simulink model "HANcoder_E407_TTA_Controller_v4_6"  (R2018b)
settings: Solver=FixedStepDiscrete  StartTime=0.0  StopTime=1  FixedStep=0.01  RelTol=1e-3
PreLoadFcn:
  | librarySetup
  | eval([bdroot,'_startup']) %Calling [modelName]_startup.m
values from neighbouring files (symbols this model uses):
  Backup_Board = 0    [HANcoder_E407_TTA_Controller_v3_5_startup.m]    (also in HANcoder_E407_TTA_Controller_v4_6_startup.m; HANcoder_E407_TTA_Controller_v4_7_startup.m; HANcoder_E407_TTA_Controller_v4_startup.m)
  basic_cycle_duration_bc0 = TM_Reset_Board   + COMP_duration    (= 212)    [HANcoder_E407_TTA_Controller_v3_5_startup.m]    (also in HANcoder_E407_TTA_Controller_v4_6_startup.m; HANcoder_E407_TTA_Controller_v4_7_startup.m; HANcoder_E407_TTA_Controller_v4_startup.m)
  basic_cycle_duration_bc1 = TM_Reset_Var_bc1 + COMP_duration    (= 288)    [HANcoder_E407_TTA_Controller_v3_5_startup.m]    (also in HANcoder_E407_TTA_Controller_v4_6_startup.m = 332; HANcoder_E407_TTA_Controller_v4_7_startup.m = 372; HANcoder_E407_TTA_Controller_v4_startup.m = 332)
  comm_delay_estimation1 = round(comm_delay_measured1*hardware_granularity/frequency_IRQ)    [HANcoder_E407_TTA_Controller_v3_5_startup.m]    (also in HANcoder_E407_TTA_Controller_v4_6_startup.m; HANcoder_E407_TTA_Controller_v4_7_startup.m; HANcoder_E407_TTA_Controller_v4_startup.m)
  comm_delay_estimation2 = round(comm_delay_measured2*hardware_granularity/frequency_IRQ)    [HANcoder_E407_TTA_Controller_v3_5_startup.m]    (also in HANcoder_E407_TTA_Controller_v4_6_startup.m; HANcoder_E407_TTA_Controller_v4_7_startup.m; HANcoder_E407_TTA_Controller_v4_startup.m)
  COMM_Period = 40    [HANcoder_E407_TTA_Controller_v3_5_startup.m]    (also in HANcoder_E407_TTA_Controller_v4_6_startup.m; HANcoder_E407_TTA_Controller_v4_7_startup.m; HANcoder_E407_TTA_Controller_v4_startup.m)
  COMM_Phase1 = Simulink.Parameter    [HANcoder_E407_TTA_Controller_v3_5_startup.m]    (also in HANcoder_E407_TTA_Controller_v4_6_startup.m; HANcoder_E407_TTA_Controller_v4_7_startup.m; HANcoder_E407_TTA_Controller_v4_startup.m)
  COMM_Phase2 = Simulink.Parameter    [HANcoder_E407_TTA_Controller_v3_5_startup.m]    (also in HANcoder_E407_TTA_Controller_v4_6_startup.m; HANcoder_E407_TTA_Controller_v4_7_startup.m; HANcoder_E407_TTA_Controller_v4_startup.m)
  COMM_Phase_init1 = Simulink.Parameter    [HANcoder_E407_TTA_Controller_v3_5_startup.m]    (also in HANcoder_E407_TTA_Controller_v4_6_startup.m; HANcoder_E407_TTA_Controller_v4_7_startup.m; HANcoder_E407_TTA_Controller_v4_startup.m)
  COMM_Phase_init2 = Simulink.Parameter    [HANcoder_E407_TTA_Controller_v3_5_startup.m]    (also in HANcoder_E407_TTA_Controller_v4_6_startup.m; HANcoder_E407_TTA_Controller_v4_7_startup.m; HANcoder_E407_TTA_Controller_v4_startup.m)
  COMP_duration = 4    [HANcoder_E407_TTA_Controller_v3_5_startup.m]    (also in HANcoder_E407_TTA_Controller_v4_6_startup.m; HANcoder_E407_TTA_Controller_v4_7_startup.m; HANcoder_E407_TTA_Controller_v4_startup.m)
  Controller1_Board = 1    [HANcoder_E407_TTA_Controller_v3_5_startup.m]    (also in HANcoder_E407_TTA_Controller_v4_6_startup.m; HANcoder_E407_TTA_Controller_v4_7_startup.m; HANcoder_E407_TTA_Controller_v4_startup.m)
  Controller2_Board = 2    [HANcoder_E407_TTA_Controller_v3_5_startup.m]    (also in HANcoder_E407_TTA_Controller_v4_6_startup.m; HANcoder_E407_TTA_Controller_v4_7_startup.m; HANcoder_E407_TTA_Controller_v4_startup.m)
  Controller3_Board = 3    [HANcoder_E407_TTA_Controller_v3_5_startup.m]    (also in HANcoder_E407_TTA_Controller_v4_6_startup.m; HANcoder_E407_TTA_Controller_v4_7_startup.m; HANcoder_E407_TTA_Controller_v4_startup.m)
  delta_a_set = Simulink.Parameter    [HANcoder_E407_TTA_Controller_v3_5_startup.m]    (also in HANcoder_E407_TTA_Controller_v4_6_startup.m; HANcoder_E407_TTA_Controller_v4_7_startup.m; HANcoder_E407_TTA_Controller_v4_startup.m)
  delta_f_set = Simulink.Parameter    [HANcoder_E407_TTA_Controller_v3_5_startup.m]    (also in HANcoder_E407_TTA_Controller_v4_6_startup.m; HANcoder_E407_TTA_Controller_v4_7_startup.m; HANcoder_E407_TTA_Controller_v4_startup.m)
  delta_max = 1    [HANcoder_E407_TTA_Controller_v3_5_startup.m]    (also in HANcoder_E407_TTA_Controller_v4_6_startup.m; HANcoder_E407_TTA_Controller_v4_7_startup.m; HANcoder_E407_TTA_Controller_v4_startup.m)
  delta_min = -1    [HANcoder_E407_TTA_Controller_v3_5_startup.m]    (also in HANcoder_E407_TTA_Controller_v4_6_startup.m; HANcoder_E407_TTA_Controller_v4_7_startup.m; HANcoder_E407_TTA_Controller_v4_startup.m)
  delta_precision = 6    [HANcoder_E407_TTA_Controller_v3_5_startup.m]    (also in HANcoder_E407_TTA_Controller_v4_6_startup.m; HANcoder_E407_TTA_Controller_v4_7_startup.m; HANcoder_E407_TTA_Controller_v4_startup.m)
  e_width = 0.1    [HANcoder_E407_TTA_Controller_v3_5_startup.m]    (also in HANcoder_E407_TTA_Controller_v4_6_startup.m; HANcoder_E407_TTA_Controller_v4_7_startup.m; HANcoder_E407_TTA_Controller_v4_startup.m)
  frequency_IRQ = 100    [HANcoder_E407_2xCAN_TEST_startup.m]    (also in HANcoder_E407_TTA_Controller_v3_5_startup.m; HANcoder_E407_TTA_Controller_v4_6_startup.m; HANcoder_E407_TTA_Controller_v4_7_startup.m; HANcoder_E407_TTA_Controller_v4_startup.m)
  HANtuneOverride = Simulink.Parameter    [HANcoder_E407_2xCAN_TEST_startup.m]    (also in HANcoder_E407_TTA_Controller_v3_5_startup.m; HANcoder_E407_TTA_Controller_v4_6_startup.m; HANcoder_E407_TTA_Controller_v4_7_startup.m; HANcoder_E407_TTA_Controller_v4_startup.m)
  hardware_granularity = 1000000    [HANcoder_E407_2xCAN_TEST_startup.m]    (also in HANcoder_E407_TTA_Controller_v3_5_startup.m; HANcoder_E407_TTA_Controller_v4_6_startup.m; HANcoder_E407_TTA_Controller_v4_7_startup.m; HANcoder_E407_TTA_Controller_v4_startup.m)
  I_a = 2.25    [HANcoder_E407_TTA_Controller_v3_5_startup.m]    (also in HANcoder_E407_TTA_Controller_v4_6_startup.m; HANcoder_E407_TTA_Controller_v4_7_startup.m; HANcoder_E407_TTA_Controller_v4_startup.m)
  I_f = 2.25    [HANcoder_E407_TTA_Controller_v3_5_startup.m]    (also in HANcoder_E407_TTA_Controller_v4_6_startup.m; HANcoder_E407_TTA_Controller_v4_7_startup.m; HANcoder_E407_TTA_Controller_v4_startup.m)
  idle_time_init = basic_cycle_duration_bc0 + basic_cycle_duration_bc1    (= 500)    [HANcoder_E407_TTA_Controller_v3_5_startup.m]    (also in HANcoder_E407_TTA_Controller_v4_6_startup.m = 544; HANcoder_E407_TTA_Controller_v4_7_startup.m = 584; HANcoder_E407_TTA_Controller_v4_startup.m = 544)
  Input_Gen_Board = 4    [HANcoder_E407_TTA_Controller_v3_5_startup.m]    (also in HANcoder_E407_TTA_Controller_v4_6_startup.m; HANcoder_E407_TTA_Controller_v4_7_startup.m; HANcoder_E407_TTA_Controller_v4_startup.m)
  LA_Clock_Gr = 1    [HANcoder_E407_TTA_Controller_v3_5_startup.m]    (also in HANcoder_E407_TTA_Controller_v4_6_startup.m; HANcoder_E407_TTA_Controller_v4_7_startup.m; HANcoder_E407_TTA_Controller_v4_startup.m)
  LA_COMM_dly = 1    [HANcoder_E407_TTA_Controller_v3_5_startup.m]    (also in HANcoder_E407_TTA_Controller_v4_6_startup.m; HANcoder_E407_TTA_Controller_v4_7_startup.m; HANcoder_E407_TTA_Controller_v4_startup.m)
  LA_COMM_Err = 1    [HANcoder_E407_TTA_Controller_v3_5_startup.m]    (also in HANcoder_E407_TTA_Controller_v4_6_startup.m; HANcoder_E407_TTA_Controller_v4_7_startup.m; HANcoder_E407_TTA_Controller_v4_startup.m)
  LA_E_Desync = 1    [HANcoder_E407_TTA_Controller_v3_5_startup.m]    (also in HANcoder_E407_TTA_Controller_v4_6_startup.m; HANcoder_E407_TTA_Controller_v4_7_startup.m; HANcoder_E407_TTA_Controller_v4_startup.m)
  LA_MEX_Flag = 1    [HANcoder_E407_TTA_Controller_v3_5_startup.m]    (also in HANcoder_E407_TTA_Controller_v4_6_startup.m; HANcoder_E407_TTA_Controller_v4_7_startup.m; HANcoder_E407_TTA_Controller_v4_startup.m)
  LA_Task_Act = 1    [HANcoder_E407_TTA_Controller_v3_5_startup.m]    (also in HANcoder_E407_TTA_Controller_v4_6_startup.m; HANcoder_E407_TTA_Controller_v4_7_startup.m; HANcoder_E407_TTA_Controller_v4_startup.m)
  m_v = 100.0    (= 100)    [HANcoder_E407_TTA_Controller_v3_5_startup.m]    (also in HANcoder_E407_TTA_Controller_v4_6_startup.m; HANcoder_E407_TTA_Controller_v4_7_startup.m; HANcoder_E407_TTA_Controller_v4_startup.m)
  Master_Role = 1    [HANcoder_E407_TTA_Controller_v3_5_startup.m]    (also in HANcoder_E407_TTA_Controller_v4_6_startup.m; HANcoder_E407_TTA_Controller_v4_7_startup.m; HANcoder_E407_TTA_Controller_v4_startup.m)
  matrix_cycle_duration = basic_cycle_duration_bc0 + basic_cycle_duration_bc1    (= 500)    [HANcoder_E407_TTA_Controller_v3_5_startup.m]    (also in HANcoder_E407_TTA_Controller_v4_6_startup.m = 544; HANcoder_E407_TTA_Controller_v4_7_startup.m = 584; HANcoder_E407_TTA_Controller_v4_startup.m = 544)
  matrix_rows = 2    [HANcoder_E407_TTA_Controller_v3_5_startup.m]    (also in HANcoder_E407_TTA_Controller_v4_6_startup.m; HANcoder_E407_TTA_Controller_v4_7_startup.m; HANcoder_E407_TTA_Controller_v4_startup.m)
  max_desync = 15    [HANcoder_E407_TTA_Controller_v3_5_startup.m]    (also in HANcoder_E407_TTA_Controller_v4_6_startup.m; HANcoder_E407_TTA_Controller_v4_7_startup.m = 30; HANcoder_E407_TTA_Controller_v4_startup.m)
  max_num_msgs_CAN1 = 2^Tx_bit_number-1    (= 7)    [HANcoder_E407_TTA_Controller_v3_5_startup.m]    (also in HANcoder_E407_TTA_Controller_v4_6_startup.m = 15; HANcoder_E407_TTA_Controller_v4_7_startup.m = 15; HANcoder_E407_TTA_Controller_v4_startup.m)
  max_num_msgs_CAN2 = max_num_msgs_CAN1    (= 7)    [HANcoder_E407_TTA_Controller_v3_5_startup.m]    (also in HANcoder_E407_TTA_Controller_v4_6_startup.m = 15; HANcoder_E407_TTA_Controller_v4_7_startup.m = 15; HANcoder_E407_TTA_Controller_v4_startup.m)
  min_desync = (-1)*max_desync    (= -15)    [HANcoder_E407_TTA_Controller_v3_5_startup.m]    (also in HANcoder_E407_TTA_Controller_v4_6_startup.m; HANcoder_E407_TTA_Controller_v4_7_startup.m = -30; HANcoder_E407_TTA_Controller_v4_startup.m)
  OutControl1_ID = 23    [HANcoder_E407_TTA_Controller_v3_5_startup.m]    (also in HANcoder_E407_TTA_Controller_v4_6_startup.m; HANcoder_E407_TTA_Controller_v4_7_startup.m; HANcoder_E407_TTA_Controller_v4_startup.m)
  OutControl2_ID = 24    [HANcoder_E407_TTA_Controller_v3_5_startup.m]    (also in HANcoder_E407_TTA_Controller_v4_6_startup.m; HANcoder_E407_TTA_Controller_v4_7_startup.m; HANcoder_E407_TTA_Controller_v4_startup.m)
  OutEmulator_ID = 25    [HANcoder_E407_TTA_Controller_v3_5_startup.m]    (also in HANcoder_E407_TTA_Controller_v4_6_startup.m = 26; HANcoder_E407_TTA_Controller_v4_7_startup.m = 26; HANcoder_E407_TTA_Controller_v4_startup.m)
  OutMaster_ID = 25    [HANcoder_E407_TTA_Controller_v4_6_startup.m]    (also in HANcoder_E407_TTA_Controller_v4_7_startup.m; HANcoder_E407_TTA_Controller_v4_startup.m = 26)
  R_al = 0.10    (= 0.1)    [HANcoder_E407_TTA_Controller_v3_5_startup.m]    (also in HANcoder_E407_TTA_Controller_v4_6_startup.m; HANcoder_E407_TTA_Controller_v4_7_startup.m; HANcoder_E407_TTA_Controller_v4_startup.m)
  R_ar = 0.10    (= 0.1)    [HANcoder_E407_TTA_Controller_v3_5_startup.m]    (also in HANcoder_E407_TTA_Controller_v4_6_startup.m; HANcoder_E407_TTA_Controller_v4_7_startup.m; HANcoder_E407_TTA_Controller_v4_startup.m)
  R_fl = 0.10    (= 0.1)    [HANcoder_E407_TTA_Controller_v3_5_startup.m]    (also in HANcoder_E407_TTA_Controller_v4_6_startup.m; HANcoder_E407_TTA_Controller_v4_7_startup.m; HANcoder_E407_TTA_Controller_v4_startup.m)
  R_fr = 0.10    (= 0.1)    [HANcoder_E407_TTA_Controller_v3_5_startup.m]    (also in HANcoder_E407_TTA_Controller_v4_6_startup.m; HANcoder_E407_TTA_Controller_v4_7_startup.m; HANcoder_E407_TTA_Controller_v4_startup.m)
  script_run = Simulink.Parameter    [HANcoder_E407_TTA_Controller_v3_5_startup.m]    (also in HANcoder_E407_TTA_Controller_v4_6_startup.m; HANcoder_E407_TTA_Controller_v4_7_startup.m; HANcoder_E407_TTA_Controller_v4_startup.m)
  SensorValues_ID = 22    [HANcoder_E407_TTA_Controller_v3_5_startup.m]    (also in HANcoder_E407_TTA_Controller_v4_6_startup.m; HANcoder_E407_TTA_Controller_v4_7_startup.m; HANcoder_E407_TTA_Controller_v4_startup.m)
  SetValues_ID = 21    [HANcoder_E407_TTA_Controller_v3_5_startup.m]    (also in HANcoder_E407_TTA_Controller_v4_6_startup.m; HANcoder_E407_TTA_Controller_v4_7_startup.m; HANcoder_E407_TTA_Controller_v4_startup.m)
  Slave_Role = 2    [HANcoder_E407_TTA_Controller_v3_5_startup.m]    (also in HANcoder_E407_TTA_Controller_v4_6_startup.m; HANcoder_E407_TTA_Controller_v4_7_startup.m; HANcoder_E407_TTA_Controller_v4_startup.m)
  speed_k_d = Simulink.Parameter    [HANcoder_E407_TTA_Controller_v3_5_startup.m]    (also in HANcoder_E407_TTA_Controller_v4_6_startup.m; HANcoder_E407_TTA_Controller_v4_7_startup.m; HANcoder_E407_TTA_Controller_v4_startup.m)
  speed_k_i = Simulink.Parameter    [HANcoder_E407_TTA_Controller_v3_5_startup.m]    (also in HANcoder_E407_TTA_Controller_v4_6_startup.m; HANcoder_E407_TTA_Controller_v4_7_startup.m; HANcoder_E407_TTA_Controller_v4_startup.m)
  speed_k_p = Simulink.Parameter    [HANcoder_E407_TTA_Controller_v3_5_startup.m]    (also in HANcoder_E407_TTA_Controller_v4_6_startup.m; HANcoder_E407_TTA_Controller_v4_7_startup.m; HANcoder_E407_TTA_Controller_v4_startup.m)
  speed_max = 10    [HANcoder_E407_TTA_Controller_v3_5_startup.m]    (also in HANcoder_E407_TTA_Controller_v4_6_startup.m; HANcoder_E407_TTA_Controller_v4_7_startup.m; HANcoder_E407_TTA_Controller_v4_startup.m)
  speed_min = -10    [HANcoder_E407_TTA_Controller_v3_5_startup.m]    (also in HANcoder_E407_TTA_Controller_v4_6_startup.m; HANcoder_E407_TTA_Controller_v4_7_startup.m; HANcoder_E407_TTA_Controller_v4_startup.m)
  speed_precision = 3    [HANcoder_E407_TTA_Controller_v3_5_startup.m]    (also in HANcoder_E407_TTA_Controller_v4_6_startup.m; HANcoder_E407_TTA_Controller_v4_7_startup.m; HANcoder_E407_TTA_Controller_v4_startup.m)
  Sync_ID = 1    [HANcoder_E407_TTA_Controller_v3_5_startup.m]    (also in HANcoder_E407_TTA_Controller_v4_6_startup.m; HANcoder_E407_TTA_Controller_v4_7_startup.m; HANcoder_E407_TTA_Controller_v4_startup.m)
  tau_max = 5    [HANcoder_E407_TTA_Controller_v3_5_startup.m]    (also in HANcoder_E407_TTA_Controller_v4_6_startup.m; HANcoder_E407_TTA_Controller_v4_7_startup.m; HANcoder_E407_TTA_Controller_v4_startup.m)
  tau_min = -5    [HANcoder_E407_TTA_Controller_v3_5_startup.m]    (also in HANcoder_E407_TTA_Controller_v4_6_startup.m; HANcoder_E407_TTA_Controller_v4_7_startup.m; HANcoder_E407_TTA_Controller_v4_startup.m)
  tau_range = abs(tau_max) + abs(tau_min)    [HANcoder_E407_TTA_Controller_v3_5_startup.m]    (also in HANcoder_E407_TTA_Controller_v4_6_startup.m; HANcoder_E407_TTA_Controller_v4_7_startup.m; HANcoder_E407_TTA_Controller_v4_startup.m)
  theta_max = (speed_max/R_fr)*matrix_cycle_duration*frequency_IRQ/hardware_granularity    (= 5)    [HANcoder_E407_TTA_Controller_v3_5_startup.m]    (also in HANcoder_E407_TTA_Controller_v4_6_startup.m = 5.44; HANcoder_E407_TTA_Controller_v4_7_startup.m = 5.84; HANcoder_E407_TTA_Controller_v4_startup.m = 5.44)
  theta_min = (-1)*theta_max    (= -5)    [HANcoder_E407_TTA_Controller_v3_5_startup.m]    (also in HANcoder_E407_TTA_Controller_v4_6_startup.m = -5.44; HANcoder_E407_TTA_Controller_v4_7_startup.m = -5.84; HANcoder_E407_TTA_Controller_v4_startup.m = -5.44)
  theta_precision = 7-(fix(log2(theta_max))+1)    [HANcoder_E407_TTA_Controller_v3_5_startup.m]    (also in HANcoder_E407_TTA_Controller_v4_6_startup.m; HANcoder_E407_TTA_Controller_v4_7_startup.m; HANcoder_E407_TTA_Controller_v4_startup.m)
  Tl_a = 0.6    [HANcoder_E407_TTA_Controller_v3_5_startup.m]    (also in HANcoder_E407_TTA_Controller_v4_6_startup.m; HANcoder_E407_TTA_Controller_v4_7_startup.m; HANcoder_E407_TTA_Controller_v4_startup.m)
  Tl_f = 0.6    [HANcoder_E407_TTA_Controller_v3_5_startup.m]    (also in HANcoder_E407_TTA_Controller_v4_6_startup.m; HANcoder_E407_TTA_Controller_v4_7_startup.m; HANcoder_E407_TTA_Controller_v4_startup.m)
  TM_Check_Output_Control1 = TM_COMM_Output_Control1 + COMM_duration    (= 188)    [HANcoder_E407_TTA_Controller_v3_5_startup.m]    (also in HANcoder_E407_TTA_Controller_v4_6_startup.m; HANcoder_E407_TTA_Controller_v4_7_startup.m; HANcoder_E407_TTA_Controller_v4_startup.m)
  TM_Check_Output_Control2 = TM_COMM_Output_Control2 + COMM_duration    (= 232)    [HANcoder_E407_TTA_Controller_v3_5_startup.m]    (also in HANcoder_E407_TTA_Controller_v4_6_startup.m; HANcoder_E407_TTA_Controller_v4_7_startup.m; HANcoder_E407_TTA_Controller_v4_startup.m)
  TM_Check_Output_Emulator = TM_COMM_Output_Emulator + COMM_duration    (= 280)    [HANcoder_E407_TTA_Controller_v3_5_startup.m]    (also in HANcoder_E407_TTA_Controller_v4_6_startup.m = 320; HANcoder_E407_TTA_Controller_v4_7_startup.m = 360; HANcoder_E407_TTA_Controller_v4_startup.m = 320)
  TM_Check_Output_Emulator_2 = TM_Check_Output_Emulator + 2    (= 282)    [HANcoder_E407_TTA_Controller_v3_5_startup.m]    (also in HANcoder_E407_TTA_Controller_v4_6_startup.m = 322; HANcoder_E407_TTA_Controller_v4_7_startup.m = 362; HANcoder_E407_TTA_Controller_v4_startup.m = 322)
  TM_Check_Output_Emulator_3 = TM_Check_Output_Emulator_2 + 2    (= 324)    [HANcoder_E407_TTA_Controller_v4_6_startup.m]    (also in HANcoder_E407_TTA_Controller_v4_7_startup.m = 364; HANcoder_E407_TTA_Controller_v4_startup.m)
  TM_Check_Sensor_Values = TM_COMM_Sensor_Values + COMM_duration    (= 132)    [HANcoder_E407_TTA_Controller_v3_5_startup.m]    (also in HANcoder_E407_TTA_Controller_v4_6_startup.m; HANcoder_E407_TTA_Controller_v4_7_startup.m; HANcoder_E407_TTA_Controller_v4_startup.m)
  TM_Check_Sensor_Values_2 = TM_Check_Sensor_Values + 2    (= 134)    [HANcoder_E407_TTA_Controller_v3_5_startup.m]    (also in HANcoder_E407_TTA_Controller_v4_6_startup.m; HANcoder_E407_TTA_Controller_v4_7_startup.m; HANcoder_E407_TTA_Controller_v4_startup.m)
  TM_Check_Set_Values = TM_COMM_Set_Values + COMM_duration    (= 88)    [HANcoder_E407_TTA_Controller_v3_5_startup.m]    (also in HANcoder_E407_TTA_Controller_v4_6_startup.m; HANcoder_E407_TTA_Controller_v4_7_startup.m; HANcoder_E407_TTA_Controller_v4_startup.m)
  TM_Check_Set_Values_2 = TM_Check_Set_Values + 2    (= 90)    [HANcoder_E407_TTA_Controller_v3_5_startup.m]    (also in HANcoder_E407_TTA_Controller_v4_6_startup.m; HANcoder_E407_TTA_Controller_v4_7_startup.m; HANcoder_E407_TTA_Controller_v4_startup.m)
  TM_Check_Sync = TM_COMM_Sync   + COMM_duration    (= 40)    [HANcoder_E407_TTA_Controller_v3_5_startup.m]    (also in HANcoder_E407_TTA_Controller_v4_6_startup.m; HANcoder_E407_TTA_Controller_v4_7_startup.m; HANcoder_E407_TTA_Controller_v4_startup.m)
  TM_Check_TOuts = TM_Count_Vote3 + COMP_duration    (= 196)    [HANcoder_E407_TTA_Controller_v3_5_startup.m]    (also in HANcoder_E407_TTA_Controller_v4_6_startup.m; HANcoder_E407_TTA_Controller_v4_7_startup.m; HANcoder_E407_TTA_Controller_v4_startup.m)
  TM_Check_Vote1 = TM_COMM_Vote1  + COMM_duration    (= 92)    [HANcoder_E407_TTA_Controller_v3_5_startup.m]    (also in HANcoder_E407_TTA_Controller_v4_6_startup.m; HANcoder_E407_TTA_Controller_v4_7_startup.m; HANcoder_E407_TTA_Controller_v4_startup.m)
  TM_Check_Vote2 = TM_COMM_Vote2  + COMM_duration    (= 140)    [HANcoder_E407_TTA_Controller_v3_5_startup.m]    (also in HANcoder_E407_TTA_Controller_v4_6_startup.m; HANcoder_E407_TTA_Controller_v4_7_startup.m; HANcoder_E407_TTA_Controller_v4_startup.m)
  TM_Check_Vote2_2 = TM_Check_Vote2 + 2    (= 142)    [HANcoder_E407_TTA_Controller_v3_5_startup.m]    (also in HANcoder_E407_TTA_Controller_v4_6_startup.m; HANcoder_E407_TTA_Controller_v4_7_startup.m; HANcoder_E407_TTA_Controller_v4_startup.m)
  TM_Check_Vote3 = TM_COMM_Vote3  + COMM_duration    (= 188)    [HANcoder_E407_TTA_Controller_v3_5_startup.m]    (also in HANcoder_E407_TTA_Controller_v4_6_startup.m; HANcoder_E407_TTA_Controller_v4_7_startup.m; HANcoder_E407_TTA_Controller_v4_startup.m)
  TM_COMM_Output_Control1 = TM_Velocity + COMP_duration    (= 148)    [HANcoder_E407_TTA_Controller_v3_5_startup.m]    (also in HANcoder_E407_TTA_Controller_v4_6_startup.m; HANcoder_E407_TTA_Controller_v4_7_startup.m; HANcoder_E407_TTA_Controller_v4_startup.m)
  TM_COMM_Output_Control2 = TM_Check_Output_Control1 + COMP_duration    (= 192)    [HANcoder_E407_TTA_Controller_v3_5_startup.m]    (also in HANcoder_E407_TTA_Controller_v4_6_startup.m; HANcoder_E407_TTA_Controller_v4_7_startup.m; HANcoder_E407_TTA_Controller_v4_startup.m)
  TM_COMM_Output_Emulator = TM_TMR + COMP_duration    (= 240)    [HANcoder_E407_TTA_Controller_v3_5_startup.m]    (also in HANcoder_E407_TTA_Controller_v4_6_startup.m = 280; HANcoder_E407_TTA_Controller_v4_7_startup.m = 320; HANcoder_E407_TTA_Controller_v4_startup.m = 280)
  TM_COMM_Output_Master = TM_Check_Output_Control2 + COMM_duration    (= 272)    [HANcoder_E407_TTA_Controller_v4_6_startup.m]    (also in HANcoder_E407_TTA_Controller_v4_7_startup.m; HANcoder_E407_TTA_Controller_v4_startup.m)
  TM_COMM_Sensor_Values = TM_Check_Set_Values + COMP_duration    (= 92)    [HANcoder_E407_TTA_Controller_v3_5_startup.m]    (also in HANcoder_E407_TTA_Controller_v4_6_startup.m; HANcoder_E407_TTA_Controller_v4_7_startup.m; HANcoder_E407_TTA_Controller_v4_startup.m)
  TM_COMM_Set_Values = TM_Update_LT + COMP_duration    (= 48)    [HANcoder_E407_TTA_Controller_v3_5_startup.m]    (also in HANcoder_E407_TTA_Controller_v4_6_startup.m; HANcoder_E407_TTA_Controller_v4_7_startup.m; HANcoder_E407_TTA_Controller_v4_startup.m)
  TM_COMM_Sync = basic_cycle_start    (= 0)    [HANcoder_E407_TTA_Controller_v3_5_startup.m]    (also in HANcoder_E407_TTA_Controller_v4_6_startup.m; HANcoder_E407_TTA_Controller_v4_7_startup.m; HANcoder_E407_TTA_Controller_v4_startup.m)
  TM_COMM_Vote1 = TM_Vote_Dec    + COMP_duration    (= 52)    [HANcoder_E407_TTA_Controller_v3_5_startup.m]    (also in HANcoder_E407_TTA_Controller_v4_6_startup.m; HANcoder_E407_TTA_Controller_v4_7_startup.m; HANcoder_E407_TTA_Controller_v4_startup.m)
  TM_COMM_Vote2 = TM_Count_Vote1 + COMP_duration    (= 100)    [HANcoder_E407_TTA_Controller_v3_5_startup.m]    (also in HANcoder_E407_TTA_Controller_v4_6_startup.m; HANcoder_E407_TTA_Controller_v4_7_startup.m; HANcoder_E407_TTA_Controller_v4_startup.m)
  TM_COMM_Vote3 = TM_Count_Vote2 + COMP_duration    (= 148)    [HANcoder_E407_TTA_Controller_v3_5_startup.m]    (also in HANcoder_E407_TTA_Controller_v4_6_startup.m; HANcoder_E407_TTA_Controller_v4_7_startup.m; HANcoder_E407_TTA_Controller_v4_startup.m)
  TM_Count_Vote1 = TM_Check_Vote1 + COMP_duration    (= 96)    [HANcoder_E407_TTA_Controller_v3_5_startup.m]    (also in HANcoder_E407_TTA_Controller_v4_6_startup.m; HANcoder_E407_TTA_Controller_v4_7_startup.m; HANcoder_E407_TTA_Controller_v4_startup.m)
  TM_Count_Vote2 = TM_Check_Vote2 + COMP_duration    (= 144)    [HANcoder_E407_TTA_Controller_v3_5_startup.m]    (also in HANcoder_E407_TTA_Controller_v4_6_startup.m; HANcoder_E407_TTA_Controller_v4_7_startup.m; HANcoder_E407_TTA_Controller_v4_startup.m)
  TM_Count_Vote3 = TM_Check_Vote3 + COMP_duration    (= 192)    [HANcoder_E407_TTA_Controller_v3_5_startup.m]    (also in HANcoder_E407_TTA_Controller_v4_6_startup.m; HANcoder_E407_TTA_Controller_v4_7_startup.m; HANcoder_E407_TTA_Controller_v4_startup.m)
  TM_Data_bc0 = TM_COMM_Sync    (= 0)    [HANcoder_E407_TTA_Controller_v3_5_startup.m]    (also in HANcoder_E407_TTA_Controller_v4_6_startup.m; HANcoder_E407_TTA_Controller_v4_7_startup.m; HANcoder_E407_TTA_Controller_v4_startup.m)
  TM_Data_bc1 = TM_Data_bc0(1:4)    [HANcoder_E407_TTA_Controller_v3_5_startup.m]    (also in HANcoder_E407_TTA_Controller_v4_6_startup.m; HANcoder_E407_TTA_Controller_v4_7_startup.m; HANcoder_E407_TTA_Controller_v4_startup.m)
  TM_New_Master = TM_Check_TOuts + COMP_duration    (= 200)    [HANcoder_E407_TTA_Controller_v3_5_startup.m]    (also in HANcoder_E407_TTA_Controller_v4_6_startup.m; HANcoder_E407_TTA_Controller_v4_7_startup.m; HANcoder_E407_TTA_Controller_v4_startup.m)
  TM_Reset_Board = TM_Reset_Var   + COMP_duration    (= 208)    [HANcoder_E407_TTA_Controller_v3_5_startup.m]    (also in HANcoder_E407_TTA_Controller_v4_6_startup.m; HANcoder_E407_TTA_Controller_v4_7_startup.m; HANcoder_E407_TTA_Controller_v4_startup.m)
  TM_Reset_Var = TM_New_Master  + COMP_duration    (= 204)    [HANcoder_E407_TTA_Controller_v3_5_startup.m]    (also in HANcoder_E407_TTA_Controller_v4_6_startup.m; HANcoder_E407_TTA_Controller_v4_7_startup.m; HANcoder_E407_TTA_Controller_v4_startup.m)
  TM_Reset_Var_bc1 = TM_Check_Output_Emulator + COMP_duration    (= 284)    [HANcoder_E407_TTA_Controller_v3_5_startup.m]    (also in HANcoder_E407_TTA_Controller_v4_6_startup.m = 328; HANcoder_E407_TTA_Controller_v4_7_startup.m = 368; HANcoder_E407_TTA_Controller_v4_startup.m = 328)
  TM_Reset_Var_bc1_2 = TM_Reset_Var_bc1 + 2    (= 286)    [HANcoder_E407_TTA_Controller_v3_5_startup.m]    (also in HANcoder_E407_TTA_Controller_v4_6_startup.m = 330; HANcoder_E407_TTA_Controller_v4_7_startup.m = 370; HANcoder_E407_TTA_Controller_v4_startup.m = 330)
  TM_Steer = TM_Check_Sensor_Values + COMP_duration    (= 136)    [HANcoder_E407_TTA_Controller_v3_5_startup.m]    (also in HANcoder_E407_TTA_Controller_v4_6_startup.m; HANcoder_E407_TTA_Controller_v4_7_startup.m; HANcoder_E407_TTA_Controller_v4_startup.m)
  TM_TMR = TM_Check_Output_Control2 + COMP_duration    (= 236)    [HANcoder_E407_TTA_Controller_v3_5_startup.m]    (also in HANcoder_E407_TTA_Controller_v4_6_startup.m = 276; HANcoder_E407_TTA_Controller_v4_7_startup.m = 316; HANcoder_E407_TTA_Controller_v4_startup.m = 276)
  TM_TMR_2 = TM_TMR + 1    (= 237)    [HANcoder_E407_TTA_Controller_v3_5_startup.m]    (also in HANcoder_E407_TTA_Controller_v4_6_startup.m = 277; HANcoder_E407_TTA_Controller_v4_7_startup.m = 317; HANcoder_E407_TTA_Controller_v4_startup.m = 277)
  TM_TMR_3 = TM_TMR + 3    (= 239)    [HANcoder_E407_TTA_Controller_v3_5_startup.m]    (also in HANcoder_E407_TTA_Controller_v4_6_startup.m = 279; HANcoder_E407_TTA_Controller_v4_7_startup.m = 319; HANcoder_E407_TTA_Controller_v4_startup.m = 279)
  TM_Torque = TM_Steer + COMP_duration    (= 140)    [HANcoder_E407_TTA_Controller_v3_5_startup.m]    (also in HANcoder_E407_TTA_Controller_v4_6_startup.m; HANcoder_E407_TTA_Controller_v4_7_startup.m; HANcoder_E407_TTA_Controller_v4_startup.m)
  TM_Type_bc0 = COMM    (= 0)    [HANcoder_E407_TTA_Controller_v3_5_startup.m]    (also in HANcoder_E407_TTA_Controller_v4_6_startup.m; HANcoder_E407_TTA_Controller_v4_7_startup.m; HANcoder_E407_TTA_Controller_v4_startup.m)
  TM_Type_bc1 = TM_Type_bc0(1:4)    [HANcoder_E407_TTA_Controller_v3_5_startup.m]    (also in HANcoder_E407_TTA_Controller_v4_6_startup.m; HANcoder_E407_TTA_Controller_v4_7_startup.m; HANcoder_E407_TTA_Controller_v4_startup.m)
  TM_Update_LT = TM_Check_Sync  + COMP_duration    (= 44)    [HANcoder_E407_TTA_Controller_v3_5_startup.m]    (also in HANcoder_E407_TTA_Controller_v4_6_startup.m; HANcoder_E407_TTA_Controller_v4_7_startup.m; HANcoder_E407_TTA_Controller_v4_startup.m)
  TM_Update_LT_2 = TM_Update_LT   + 2    (= 46)    [HANcoder_E407_TTA_Controller_v3_5_startup.m]    (also in HANcoder_E407_TTA_Controller_v4_6_startup.m; HANcoder_E407_TTA_Controller_v4_7_startup.m; HANcoder_E407_TTA_Controller_v4_startup.m)
  TM_Velocity = TM_Torque + COMP_duration    (= 144)    [HANcoder_E407_TTA_Controller_v3_5_startup.m]    (also in HANcoder_E407_TTA_Controller_v4_6_startup.m; HANcoder_E407_TTA_Controller_v4_7_startup.m; HANcoder_E407_TTA_Controller_v4_startup.m)
  TM_Vote_Dec = TM_Update_LT   + COMP_duration    (= 48)    [HANcoder_E407_TTA_Controller_v3_5_startup.m]    (also in HANcoder_E407_TTA_Controller_v4_6_startup.m; HANcoder_E407_TTA_Controller_v4_7_startup.m; HANcoder_E407_TTA_Controller_v4_startup.m)
  TM_Vote_Dec_2 = TM_Vote_Dec    + 2    (= 50)    [HANcoder_E407_TTA_Controller_v3_5_startup.m]    (also in HANcoder_E407_TTA_Controller_v4_6_startup.m; HANcoder_E407_TTA_Controller_v4_7_startup.m; HANcoder_E407_TTA_Controller_v4_startup.m)
  torque_a_k_d = Simulink.Parameter    [HANcoder_E407_TTA_Controller_v3_5_startup.m]    (also in HANcoder_E407_TTA_Controller_v4_6_startup.m; HANcoder_E407_TTA_Controller_v4_7_startup.m; HANcoder_E407_TTA_Controller_v4_startup.m)
  torque_a_k_i = Simulink.Parameter    [HANcoder_E407_TTA_Controller_v3_5_startup.m]    (also in HANcoder_E407_TTA_Controller_v4_6_startup.m; HANcoder_E407_TTA_Controller_v4_7_startup.m; HANcoder_E407_TTA_Controller_v4_startup.m)
  torque_a_k_p = Simulink.Parameter    [HANcoder_E407_TTA_Controller_v3_5_startup.m]    (also in HANcoder_E407_TTA_Controller_v4_6_startup.m; HANcoder_E407_TTA_Controller_v4_7_startup.m; HANcoder_E407_TTA_Controller_v4_startup.m)
  torque_f_k_d = Simulink.Parameter    [HANcoder_E407_TTA_Controller_v3_5_startup.m]    (also in HANcoder_E407_TTA_Controller_v4_6_startup.m; HANcoder_E407_TTA_Controller_v4_7_startup.m; HANcoder_E407_TTA_Controller_v4_startup.m)
  torque_f_k_i = Simulink.Parameter    [HANcoder_E407_TTA_Controller_v3_5_startup.m]    (also in HANcoder_E407_TTA_Controller_v4_6_startup.m; HANcoder_E407_TTA_Controller_v4_7_startup.m; HANcoder_E407_TTA_Controller_v4_startup.m)
  ... (+7 more)
undefined symbols (not defined in the file or in its folder): A0, A1, A2, A3, A4, CON2, CON3, CON4, D10, D12, D13, D2, D3, D8, D9
libraries: hdlsllib x467, HANcoder_STM32_Target x30, simulink x3, simulink_extras x1
(part 6 of 80)

== system HANcoder_E407_TTA_Controller_v4_6/HANcoder STM32 Target - E407-STM32 algorithm/TTA CAN System/TTA System/Matrix Cycle Manager ==
  note: Backup Board
  note: Input generator board condition
  note: Controller boards condition
  note: Output Send_Message
      | Send: 1
      | Do not send: 0
  note: Output Receive_Message
      | Receive: 1
      | Do not receive: 0
  note: Output Receive_Message
      | Receive: 1
      | Do not receive: 0
  note: Output Send_Message
      | Send: 1
      | Do not send: 0
  note: Vehicle emulator board condition
  note: Backup board condition
  Enable : EnablePort  PropagateVarSize=During execution
  Backup Board Matrix Cycle : Subsystem  Commented=on
  Bus Selector : BusSelector  OutputSignals=signal1,signal2,signal3,signal4
  Bus Creator : BusCreator  Inputs=4
  Bus Creator1 : BusCreator  Inputs=4
  Bus Creator2 : BusCreator  Inputs=4
  Bus Creator3 : BusCreator  Commented=on  Inputs=4
  Constant : Constant  Value=Controller1_Board
  Constant1 : Constant  Value=Controller2_Board
  Constant2 : Constant  Value=Controller3_Board
  Constant3 : Constant  Value=Input_Gen_Board
  Constant4 : Constant  Value=Vehicle_Em_Board
  Constant5 : Constant  Commented=on  Value=Backup_Board
  Controller Matrix Cycle : Subsystem
  Data Store Read : DataStoreRead  DataStoreName=Board_ID
  Data Store Read10 : DataStoreRead  DataStoreName=basic_cycle_count
  Equal{,1..4} (5 alike) : RelationalOperator  Operator===  OutDataTypeStr=boolean  RndMeth=Simplest
  Equal5 : RelationalOperator  Commented=on  Operator===  OutDataTypeStr=boolean  RndMeth=Simplest
  Input Generator Matrix Cycle : Subsystem
  OR : Logic  Operator=OR  Inputs=3  IconShape=distinctive  AllPortsSameDT=off  OutDataTypeStr=boolean
  Switch : Switch  Criteria=u2 > Threshold
  Switch1 : Switch  Criteria=u2 > Threshold
  Switch2 : Switch  Criteria=u2 > Threshold
  Vehicle Emulator Matrix Cycle : Subsystem
  Send_Message_CAN1 : Outport  OutputWhenDisabled=reset  InitialOutput=0
  Send_Message_CAN2 : Outport  Port=2  OutputWhenDisabled=reset  InitialOutput=0
  Receive_Message_CAN1 : Outport  Port=3  OutputWhenDisabled=reset  InitialOutput=0
  Receive_Message_CAN2 : Outport  Port=4  OutputWhenDisabled=reset  InitialOutput=0
  wires:
  Data Store Read10/1 -> Input Generator Matrix Cycle/1(basic_cycle), Backup Board Matrix Cycle/1(basic_cycle), Vehicle Emulator Matrix Cycle/1(basic_cycle), Controller Matrix Cycle/1(basic_cycle)
  Constant/1 -> Equal/2
  Constant1/1 -> Equal1/2
  Constant2/1 -> Equal2/2
  Equal/1 -> OR/1
  Equal1/1 -> OR/2
  Equal2/1 -> OR/3
  OR/1 -> Switch1/2, Controller Matrix Cycle/Enable
  Constant3/1 -> Equal3/2
  Equal3/1 -> Input Generator Matrix Cycle/Enable, Switch/2
  Constant4/1 -> Equal4/2
  Equal4/1 -> Switch2/2, Vehicle Emulator Matrix Cycle/Enable
  Controller Matrix Cycle/1(Send_CAN1) -> Bus Creator/1
  Controller Matrix Cycle/2(Send_CAN2) -> Bus Creator/2
  Controller Matrix Cycle/3(Receive_CAN1) -> Bus Creator/3
  Controller Matrix Cycle/4(Receive_CAN2) -> Bus Creator/4
  Input Generator Matrix Cycle/1(Send_CAN1) -> Bus Creator1/1
  Input Generator Matrix Cycle/2(Send_CAN2) -> Bus Creator1/2
  Input Generator Matrix Cycle/3(Receive_CAN1) -> Bus Creator1/3
  Input Generator Matrix Cycle/4(Receive_CAN2) -> Bus Creator1/4
  Vehicle Emulator Matrix Cycle/1(Send_CAN1) -> Bus Creator2/1
  Vehicle Emulator Matrix Cycle/2(Send_CAN2) -> Bus Creator2/2
  Vehicle Emulator Matrix Cycle/3(Receive_CAN1) -> Bus Creator2/3
  Vehicle Emulator Matrix Cycle/4(Receive_CAN2) -> Bus Creator2/4
  Bus Creator2/1 -> Switch2/1
  Bus Creator1/1 -> Switch/1
  Bus Creator/1 -> Switch1/1
  Switch/1 -> Switch1/3
  Switch1/1 -> Bus Selector/1
  Bus Selector/4 -> Receive_Message_CAN2/1  "<signal4>"
  Bus Selector/3 -> Receive_Message_CAN1/1  "<signal3>"
  Bus Selector/2 -> Send_Message_CAN2/1  "<signal2>"
  Bus Selector/1 -> Send_Message_CAN1/1  "<signal1>"
  Equal5/1 -> Backup Board Matrix Cycle/Enable
  Constant5/1 -> Equal5/2
  Data Store Read/1 -> Equal5/1, Equal4/1, Equal3/1, Equal2/1, Equal1/1, Equal/1
  Backup Board Matrix Cycle/4(Receive_CAN2) -> Bus Creator3/4
  Backup Board Matrix Cycle/3(Receive_CAN1) -> Bus Creator3/3
  Bus Creator3/1 -> Switch2/3
  Backup Board Matrix Cycle/1(Send_CAN1) -> Bus Creator3/1
  Backup Board Matrix Cycle/2(Send_CAN2) -> Bus Creator3/2
  Switch2/1 -> Switch/3

== system HANcoder_E407_TTA_Controller_v4_6/HANcoder STM32 Target - E407-STM32 algorithm/TTA CAN System/CAN1 Recieve/RxID_CAN/OutControl1_ID_CAN ==
  Enable : EnablePort
  CAN receive1 : Subsystem  Tag=HANcoder_TARGET_STM32_E407  AncestorBlock=HANcoder_STM32_Target/STM32-E407/CAN/CAN/CAN receive  mask(CAN receive){canBus=CAN 1, outputNumber=8, dataType=uint8, byteOrder=off, tsamp=-1}
      mask prompts: canBus "CAN channel"; outputNumber "Output ports"; dataType "Output datatype"; byteOrder "Byte order: Checked = MSB first, unchecked = LSB first."; tsamp "Sample time"
      mask help:
      | Function
      | ==========
      | Receive the newest message from the specified CAN channel.
      |
      | Parameters
      | ==========
      | CAN channel:             The CAN channel to send the message on.
      | Output ports:             The amount of output ports
      | Output datatype:       The datatype of the output ports
      | Byte order:                 Select MSB or LSB first
      | Sample time:              -1 or divisible by base sample time [seconds]
      |
      | Input
      | ==========
      | Port 1:                       CAN ID(uint32) in hexadecimal ie: hex2dec('0a')
      |
      | Output
      | ==========
      | Port 1:                       Checks for new message(int8)
      | Port 2..9                     Message data
      mask init:
      | sfcn_can_receive_mcb(canBus, outputNumber, dataType, byteOrder)
      settings: MoveFcn=drawLogos
      mask Help: web('sfcn_can_receive.html');
      mask TypeOptions canBus: CAN 1 | CAN 2
      mask TypeOptions dataType: int8 | uint8 | int16 | uint16 | int32 | uint32 | boolean
      mask Display:
      | fprintf('Receive on\nCAN %x', canBus);
      | port_label('output', 1, 'new');
      | port_label('input', 1, 'ID');patch([135 141 141],[8 14 2],[1 0 0]);patch([143 143 149],[14 2 8],[0 0 0.35]);
  Constant6 : Constant  Value=OutControl1_ID  OutDataTypeStr=uint32
  CAN_new : Outport  OutputWhenDisabled=reset  InitialOutput=0
  Out2 : Outport  Port=2  OutputWhenDisabled=reset  InitialOutput=0
  Out3 : Outport  Port=3  OutputWhenDisabled=reset  InitialOutput=0
  Out4 : Outport  Port=4  OutputWhenDisabled=reset  InitialOutput=0
  Out5 : Outport  Port=5  OutputWhenDisabled=reset  InitialOutput=0
  Out6 : Outport  Port=6  OutputWhenDisabled=reset  InitialOutput=0
  Out7 : Outport  Port=7  OutputWhenDisabled=reset  InitialOutput=0
  Out8 : Outport  Port=8  OutputWhenDisabled=reset  InitialOutput=0
  Out9 : Outport  Port=9  OutputWhenDisabled=reset  InitialOutput=0
  wires:
  CAN receive1/1(Out1) -> CAN_new/1
  CAN receive1/8(Out8) -> Out8/1
  CAN receive1/3(Out3) -> Out3/1
  CAN receive1/2(Out2) -> Out2/1
  CAN receive1/6(Out6) -> Out6/1
  CAN receive1/7(Out7) -> Out7/1
  CAN receive1/4(Out4) -> Out4/1
  CAN receive1/5(Out5) -> Out5/1
  CAN receive1/9(Out9) -> Out9/1
  Constant6/1 -> CAN receive1/1(In1)

== system HANcoder_E407_TTA_Controller_v4_6/HANcoder STM32 Target - E407-STM32 algorithm/TTA CAN System/CAN1 Recieve/RxID_CAN/OutControl2_ID_CAN ==
  Enable : EnablePort
  CAN receive1 : Subsystem  Tag=HANcoder_TARGET_STM32_E407  AncestorBlock=HANcoder_STM32_Target/STM32-E407/CAN/CAN/CAN receive  mask(CAN receive){canBus=CAN 1, outputNumber=8, dataType=uint8, byteOrder=off, tsamp=-1}
      mask prompts: canBus "CAN channel"; outputNumber "Output ports"; dataType "Output datatype"; byteOrder "Byte order: Checked = MSB first, unchecked = LSB first."; tsamp "Sample time"
      mask help:
      | Function
      | ==========
      | Receive the newest message from the specified CAN channel.
      |
      | Parameters
      | ==========
      | CAN channel:             The CAN channel to send the message on.
      | Output ports:             The amount of output ports
      | Output datatype:       The datatype of the output ports
      | Byte order:                 Select MSB or LSB first
      | Sample time:              -1 or divisible by base sample time [seconds]
      |
      | Input
      | ==========
      | Port 1:                       CAN ID(uint32) in hexadecimal ie: hex2dec('0a')
      |
      | Output
      | ==========
      | Port 1:                       Checks for new message(int8)
      | Port 2..9                     Message data
      mask init:
      | sfcn_can_receive_mcb(canBus, outputNumber, dataType, byteOrder)
      settings: MoveFcn=drawLogos
      mask Help: web('sfcn_can_receive.html');
      mask TypeOptions canBus: CAN 1 | CAN 2
      mask TypeOptions dataType: int8 | uint8 | int16 | uint16 | int32 | uint32 | boolean
      mask Display:
      | fprintf('Receive on\nCAN %x', canBus);
      | port_label('output', 1, 'new');
      | port_label('input', 1, 'ID');patch([135 141 141],[8 14 2],[1 0 0]);patch([143 143 149],[14 2 8],[0 0 0.35]);
  Constant7 : Constant  Value=OutControl2_ID  OutDataTypeStr=uint32
  CAN_new : Outport  OutputWhenDisabled=reset  InitialOutput=0
  Out2 : Outport  Port=2  OutputWhenDisabled=reset  InitialOutput=0
  Out3 : Outport  Port=3  OutputWhenDisabled=reset  InitialOutput=0
  Out4 : Outport  Port=4  OutputWhenDisabled=reset  InitialOutput=0
  Out5 : Outport  Port=5  OutputWhenDisabled=reset  InitialOutput=0
  Out6 : Outport  Port=6  OutputWhenDisabled=reset  InitialOutput=0
  Out7 : Outport  Port=7  OutputWhenDisabled=reset  InitialOutput=0
  Out8 : Outport  Port=8  OutputWhenDisabled=reset  InitialOutput=0
  Out9 : Outport  Port=9  OutputWhenDisabled=reset  InitialOutput=0
  wires:
  Constant7/1 -> CAN receive1/1(In1)
  CAN receive1/9(Out9) -> Out9/1
  CAN receive1/5(Out5) -> Out5/1
  CAN receive1/4(Out4) -> Out4/1
  CAN receive1/7(Out7) -> Out7/1
  CAN receive1/6(Out6) -> Out6/1
  CAN receive1/2(Out2) -> Out2/1
  CAN receive1/3(Out3) -> Out3/1
  CAN receive1/8(Out8) -> Out8/1
  CAN receive1/1(Out1) -> CAN_new/1

== system HANcoder_E407_TTA_Controller_v4_6/HANcoder STM32 Target - E407-STM32 algorithm/TTA CAN System/CAN1 Recieve/RxID_CAN/OutEmulator_ID_CAN ==
  Enable : EnablePort
  CAN receive1 : Subsystem  Tag=HANcoder_TARGET_STM32_E407  AncestorBlock=HANcoder_STM32_Target/STM32-E407/CAN/CAN/CAN receive  mask(CAN receive){canBus=CAN 1, outputNumber=8, dataType=uint8, byteOrder=off, tsamp=-1}
      mask prompts: canBus "CAN channel"; outputNumber "Output ports"; dataType "Output datatype"; byteOrder "Byte order: Checked = MSB first, unchecked = LSB first."; tsamp "Sample time"
      mask help:
      | Function
      | ==========
      | Receive the newest message from the specified CAN channel.
      |
      | Parameters
      | ==========
      | CAN channel:             The CAN channel to send the message on.
      | Output ports:             The amount of output ports
      | Output datatype:       The datatype of the output ports
      | Byte order:                 Select MSB or LSB first
      | Sample time:              -1 or divisible by base sample time [seconds]
      |
      | Input
      | ==========
      | Port 1:                       CAN ID(uint32) in hexadecimal ie: hex2dec('0a')
      |
      | Output
      | ==========
      | Port 1:                       Checks for new message(int8)
      | Port 2..9                     Message data
      mask init:
      | sfcn_can_receive_mcb(canBus, outputNumber, dataType, byteOrder)
      settings: MoveFcn=drawLogos
      mask Help: web('sfcn_can_receive.html');
      mask TypeOptions canBus: CAN 1 | CAN 2
      mask TypeOptions dataType: int8 | uint8 | int16 | uint16 | int32 | uint32 | boolean
      mask Display:
      | fprintf('Receive on\nCAN %x', canBus);
      | port_label('output', 1, 'new');
      | port_label('input', 1, 'ID');patch([135 141 141],[8 14 2],[1 0 0]);patch([143 143 149],[14 2 8],[0 0 0.35]);
  Constant8 : Constant  Value=OutEmulator_ID  OutDataTypeStr=uint32
  CAN_new : Outport  OutputWhenDisabled=reset  InitialOutput=0
  Out2 : Outport  Port=2  OutputWhenDisabled=reset  InitialOutput=0
  Out3 : Outport  Port=3  OutputWhenDisabled=reset  InitialOutput=0
  Out4 : Outport  Port=4  OutputWhenDisabled=reset  InitialOutput=0
  Out5 : Outport  Port=5  OutputWhenDisabled=reset  InitialOutput=0
  Out6 : Outport  Port=6  OutputWhenDisabled=reset  InitialOutput=0
  Out7 : Outport  Port=7  OutputWhenDisabled=reset  InitialOutput=0
  Out8 : Outport  Port=8  OutputWhenDisabled=reset  InitialOutput=0
  Out9 : Outport  Port=9  OutputWhenDisabled=reset  InitialOutput=0
  wires:
  CAN receive1/1(Out1) -> CAN_new/1
  CAN receive1/8(Out8) -> Out8/1
  CAN receive1/3(Out3) -> Out3/1
  CAN receive1/2(Out2) -> Out2/1
  CAN receive1/6(Out6) -> Out6/1
  CAN receive1/7(Out7) -> Out7/1
  CAN receive1/4(Out4) -> Out4/1
  CAN receive1/5(Out5) -> Out5/1
  CAN receive1/9(Out9) -> Out9/1
  Constant8/1 -> CAN receive1/1(In1)

== system HANcoder_E407_TTA_Controller_v4_6/HANcoder STM32 Target - E407-STM32 algorithm/TTA CAN System/CAN1 Recieve/RxID_CAN/SensorValues_ID_CAN ==
  Enable : EnablePort
  CAN receive1 : Subsystem  Tag=HANcoder_TARGET_STM32_E407  AncestorBlock=HANcoder_STM32_Target/STM32-E407/CAN/CAN/CAN receive  mask(CAN receive){canBus=CAN 1, outputNumber=8, dataType=uint8, byteOrder=off, tsamp=-1}
      mask prompts: canBus "CAN channel"; outputNumber "Output ports"; dataType "Output datatype"; byteOrder "Byte order: Checked = MSB first, unchecked = LSB first."; tsamp "Sample time"
      mask help:
      | Function
      | ==========
      | Receive the newest message from the specified CAN channel.
      |
      | Parameters
      | ==========
      | CAN channel:             The CAN channel to send the message on.
      | Output ports:             The amount of output ports
      | Output datatype:       The datatype of the output ports
      | Byte order:                 Select MSB or LSB first
      | Sample time:              -1 or divisible by base sample time [seconds]
      |
      | Input
      | ==========
      | Port 1:                       CAN ID(uint32) in hexadecimal ie: hex2dec('0a')
      |
      | Output
      | ==========
      | Port 1:                       Checks for new message(int8)
      | Port 2..9                     Message data
      mask init:
      | sfcn_can_receive_mcb(canBus, outputNumber, dataType, byteOrder)
      settings: MoveFcn=drawLogos
      mask Help: web('sfcn_can_receive.html');
      mask TypeOptions canBus: CAN 1 | CAN 2
      mask TypeOptions dataType: int8 | uint8 | int16 | uint16 | int32 | uint32 | boolean
      mask Display:
      | fprintf('Receive on\nCAN %x', canBus);
      | port_label('output', 1, 'new');
      | port_label('input', 1, 'ID');patch([135 141 141],[8 14 2],[1 0 0]);patch([143 143 149],[14 2 8],[0 0 0.35]);
  Constant5 : Constant  Value=SensorValues_ID  OutDataTypeStr=uint32
  CAN_new : Outport  OutputWhenDisabled=reset  InitialOutput=0
  Out2 : Outport  Port=2  OutputWhenDisabled=reset  InitialOutput=0
  Out3 : Outport  Port=3  OutputWhenDisabled=reset  InitialOutput=0
  Out4 : Outport  Port=4  OutputWhenDisabled=reset  InitialOutput=0
  Out5 : Outport  Port=5  OutputWhenDisabled=reset  InitialOutput=0
  Out6 : Outport  Port=6  OutputWhenDisabled=reset  InitialOutput=0
  Out7 : Outport  Port=7  OutputWhenDisabled=reset  InitialOutput=0
  Out8 : Outport  Port=8  OutputWhenDisabled=reset  InitialOutput=0
  Out9 : Outport  Port=9  OutputWhenDisabled=reset  InitialOutput=0
  wires:
  Constant5/1 -> CAN receive1/1(In1)
  CAN receive1/9(Out9) -> Out9/1
  CAN receive1/5(Out5) -> Out5/1
  CAN receive1/4(Out4) -> Out4/1
  CAN receive1/7(Out7) -> Out7/1
  CAN receive1/6(Out6) -> Out6/1
  CAN receive1/2(Out2) -> Out2/1
  CAN receive1/3(Out3) -> Out3/1
  CAN receive1/8(Out8) -> Out8/1
  CAN receive1/1(Out1) -> CAN_new/1

== system HANcoder_E407_TTA_Controller_v4_6/HANcoder STM32 Target - E407-STM32 algorithm/TTA CAN System/CAN1 Recieve/RxID_CAN/SetValues_ID_CAN ==
  Enable : EnablePort
  CAN receive1 : Subsystem  Tag=HANcoder_TARGET_STM32_E407  AncestorBlock=HANcoder_STM32_Target/STM32-E407/CAN/CAN/CAN receive  mask(CAN receive){canBus=CAN 1, outputNumber=8, dataType=uint8, byteOrder=off, tsamp=-1}
      mask prompts: canBus "CAN channel"; outputNumber "Output ports"; dataType "Output datatype"; byteOrder "Byte order: Checked = MSB first, unchecked = LSB first."; tsamp "Sample time"
      mask help:
      | Function
      | ==========
      | Receive the newest message from the specified CAN channel.
      |
      | Parameters
      | ==========
      | CAN channel:             The CAN channel to send the message on.
      | Output ports:             The amount of output ports
      | Output datatype:       The datatype of the output ports
      | Byte order:                 Select MSB or LSB first
      | Sample time:              -1 or divisible by base sample time [seconds]
      |
      | Input
      | ==========
      | Port 1:                       CAN ID(uint32) in hexadecimal ie: hex2dec('0a')
      |
      | Output
      | ==========
      | Port 1:                       Checks for new message(int8)
      | Port 2..9                     Message data
      mask init:
      | sfcn_can_receive_mcb(canBus, outputNumber, dataType, byteOrder)
      settings: MoveFcn=drawLogos
      mask Help: web('sfcn_can_receive.html');
      mask TypeOptions canBus: CAN 1 | CAN 2
      mask TypeOptions dataType: int8 | uint8 | int16 | uint16 | int32 | uint32 | boolean
      mask Display:
      | fprintf('Receive on\nCAN %x', canBus);
      | port_label('output', 1, 'new');
      | port_label('input', 1, 'ID');patch([135 141 141],[8 14 2],[1 0 0]);patch([143 143 149],[14 2 8],[0 0 0.35]);
  Constant4 : Constant  Value=SetValues_ID  OutDataTypeStr=uint32
  CAN_new : Outport  OutputWhenDisabled=reset  InitialOutput=0
  Out2 : Outport  Port=2  OutputWhenDisabled=reset  InitialOutput=0
  Out3 : Outport  Port=3  OutputWhenDisabled=reset  InitialOutput=0
  Out4 : Outport  Port=4  OutputWhenDisabled=reset  InitialOutput=0
  Out5 : Outport  Port=5  OutputWhenDisabled=reset  InitialOutput=0
  Out6 : Outport  Port=6  OutputWhenDisabled=reset  InitialOutput=0
  Out7 : Outport  Port=7  OutputWhenDisabled=reset  InitialOutput=0
  Out8 : Outport  Port=8  OutputWhenDisabled=reset  InitialOutput=0
  Out9 : Outport  Port=9  OutputWhenDisabled=reset  InitialOutput=0
  wires:
  CAN receive1/1(Out1) -> CAN_new/1
  CAN receive1/8(Out8) -> Out8/1
  CAN receive1/3(Out3) -> Out3/1
  CAN receive1/2(Out2) -> Out2/1
  CAN receive1/6(Out6) -> Out6/1
  CAN receive1/7(Out7) -> Out7/1
  CAN receive1/4(Out4) -> Out4/1
  CAN receive1/5(Out5) -> Out5/1
  CAN receive1/9(Out9) -> Out9/1
  Constant4/1 -> CAN receive1/1(In1)

== system HANcoder_E407_TTA_Controller_v4_6/HANcoder STM32 Target - E407-STM32 algorithm/TTA CAN System/CAN1 Recieve/RxID_CAN/Sync_ID_CAN ==
  Enable : EnablePort
  CAN receive1 : Subsystem  Tag=HANcoder_TARGET_STM32_E407  AncestorBlock=HANcoder_STM32_Target/STM32-E407/CAN/CAN/CAN receive  mask(CAN receive){canBus=CAN 1, outputNumber=8, dataType=uint8, byteOrder=off, tsamp=-1}
      mask prompts: canBus "CAN channel"; outputNumber "Output ports"; dataType "Output datatype"; byteOrder "Byte order: Checked = MSB first, unchecked = LSB first."; tsamp "Sample time"
      mask help:
      | Function
      | ==========
      | Receive the newest message from the specified CAN channel.
      |
      | Parameters
      | ==========
      | CAN channel:             The CAN channel to send the message on.
      | Output ports:             The amount of output ports
      | Output datatype:       The datatype of the output ports
      | Byte order:                 Select MSB or LSB first
      | Sample time:              -1 or divisible by base sample time [seconds]
      |
      | Input
      | ==========
      | Port 1:                       CAN ID(uint32) in hexadecimal ie: hex2dec('0a')
      |
      | Output
      | ==========
      | Port 1:                       Checks for new message(int8)
      | Port 2..9                     Message data
      mask init:
      | sfcn_can_receive_mcb(canBus, outputNumber, dataType, byteOrder)
      settings: MoveFcn=drawLogos
      mask Help: web('sfcn_can_receive.html');
      mask TypeOptions canBus: CAN 1 | CAN 2
      mask TypeOptions dataType: int8 | uint8 | int16 | uint16 | int32 | uint32 | boolean
      mask Display:
      | fprintf('Receive on\nCAN %x', canBus);
      | port_label('output', 1, 'new');
      | port_label('input', 1, 'ID');patch([135 141 141],[8 14 2],[1 0 0]);patch([143 143 149],[14 2 8],[0 0 0.35]);
  Constant : Constant  Value=Sync_ID  OutDataTypeStr=uint32
  CAN_new : Outport  OutputWhenDisabled=reset  InitialOutput=0
  Out2 : Outport  Port=2  OutputWhenDisabled=reset  InitialOutput=0
  Out3 : Outport  Port=3  OutputWhenDisabled=reset  InitialOutput=0
  Out4 : Outport  Port=4  OutputWhenDisabled=reset  InitialOutput=0
  Out5 : Outport  Port=5  OutputWhenDisabled=reset  InitialOutput=0
  Out6 : Outport  Port=6  OutputWhenDisabled=reset  InitialOutput=0
  Out7 : Outport  Port=7  OutputWhenDisabled=reset  InitialOutput=0
  Out8 : Outport  Port=8  OutputWhenDisabled=reset  InitialOutput=0
  Out9 : Outport  Port=9  OutputWhenDisabled=reset  InitialOutput=0
  wires:
  CAN receive1/1(Out1) -> CAN_new/1
  CAN receive1/8(Out8) -> Out8/1
  CAN receive1/3(Out3) -> Out3/1
  CAN receive1/2(Out2) -> Out2/1
  CAN receive1/6(Out6) -> Out6/1
  CAN receive1/7(Out7) -> Out7/1
  CAN receive1/4(Out4) -> Out4/1
  CAN receive1/5(Out5) -> Out5/1
  CAN receive1/9(Out9) -> Out9/1
  Constant/1 -> CAN receive1/1(In1)
